simulink model "testIntegrator"  (Simulink 7.4)
settings: Solver=ode45  StartTime=0.0  StopTime=10.0  RelTol=1e-3
libraries: BLOM_Lib x1
settings Model: Creator=Kyle  LastModifiedBy=Kyle

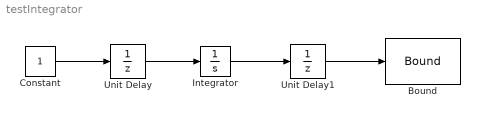
== system testIntegrator ==
  Bound : BLOM_Lib/Bound  SystemSampleTime=-1  ub=inf  lb=-inf  initial_step=on  intermediate_step=off  final_step=off
  Constant : Constant  OutDataType=fixdt(1, 16)  OutScaling=2^0
  Integrator : Integrator
  Unit Delay : UnitDelay  SampleTime=-1
  Unit Delay1 : UnitDelay  SampleTime=-1
  wires:
  Constant/1 -> Unit Delay/1
  Unit Delay/1 -> Integrator/1
  Integrator/1 -> Unit Delay1/1
  Unit Delay1/1 -> Bound/1
